simulink library "speedgoatlib_fpga_analog_io"  (R2024b)
settings: Solver=VariableStepAuto  StartTime=0.0  StopTime=10.0  RelTol=1e-3
undefined symbols (not defined in the file): IO336, sg_fpga_callBackInit_m_a1, sg_fpga_io324_analog_input_m, sg_fpga_io324_analog_output_m, sg_fpga_io324_analog_setup_m, sg_fpga_io325_analog_input_m, sg_fpga_io325_analog_output_m, sg_fpga_io325_analog_setup_m, sg_fpga_io334_analog_input_m, sg_fpga_io334_analog_output_m, sg_fpga_io334_analog_setup_m, sg_fpga_io336_analog_input_m, sg_fpga_io336_analog_output_m, sg_fpga_io336_analog_setup_m, sg_fpga_io337_analog_input_m, sg_fpga_io337_analog_output_m, sg_fpga_io337_analog_setup_m, sg_fpga_io3xx_120_analog_input_m, sg_fpga_io3xx_120_analog_output_m, sg_fpga_io3xx_120_analog_setup_m
(part 3 of 4)

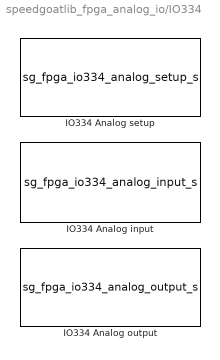
== system speedgoatlib_fpga_analog_io/IO334 ==
  IO334 Analog input : S-Function  InitFcn=sg_fpga_io334_analog_input_m.runInitFcn();  FunctionName=sg_fpga_io334_analog_input_s  Parameters=id, parSampleTime, parAiChannels, parAiChannelsStreamed, parAiReadPrevValue, parAiEnableFrame, parAiFrameSize  SFunctionDeploymentMode=off  EnableBusSupport=off  mask(ad_fpga_IO334){id=1, parSampleTime=-1, pciSlot=[-1,-1], parAiChannels=[1 2], parAiChannelsStreamed=[1 2], parAiReadPrevValue=0, parAiEnableFrame=0, parAdcCoupling=[1 1 1 1], parAdcContSampling=0, parAdcDmaEnable=0, parAdcActiveDmaDevices=[1 1 1 1], parAiFrameSize=100}
      mask prompts: id "Configurable I/O Module ID"; parSampleTime "Sample Time [s]"
      mask help: Speedgoat Driver Block<br>IO334-325k - IO334 Analog Input<br><br>&copy; 2007 - 2026, Speedgoat GmbH, <a href="matlab: web('www.speedgoat.com','-browser');">www.speedgoat.com</a>
      mask init:
      | sg_fpga_io334_analog_input_m.runMaskInit();
      mask Help: eval('sg.utils.help.show(''io_main/refentry_io334_analog_input_v1'');')
      mask TypeOptions id: 1 | 2 | 3 | 4 | 5 | 6 | 7 | 8 | 9 | 10
      mask Display: disp('Speedgoat\nIO334-325k\nAnalog input v1\nModule ID: 1');port_label('output',1,'1');port_label('output',2,'2');
  IO334 Analog output : S-Function  InitFcn=sg_fpga_io334_analog_output_m.runInitFcn();  FunctionName=sg_fpga_io334_analog_output_s  Parameters=id, parSampleTime, parAoChannels, parAoVoltageRange, parAoInitValues, parAoReset, parAoEnableFrame, parAoFrameSize  SFunctionDeploymentMode=off  EnableBusSupport=off  mask(da_fpga_IO334){id=1, parSampleTime=-1, pciSlot=[-1,-1], board=IO336-325k, parAoChannels=[1 3 5], parAoVoltageRange=[1 1 1], parDacOverRange=[0 0 0 0 0 0 0 0], parAoInitValues=[0 0 0], parAoReset=[1 1 1], parDacSyncOut=1, parAoEnableFrame=1, parDacActiveDmaDevices=[1 1 1 1], parDacDmaLatency=2, parAoFrameSize=1000}
      mask prompts: id "Configurable I/O Module ID"; parSampleTime "Sample Time [s]"
      mask help: Speedgoat Driver Block<br>IO334-325k - IO334 Analog Output<br><br>&copy; 2007 - 2026, Speedgoat GmbH, <a href="matlab: web('www.speedgoat.com','-browser');">www.speedgoat.com</a>
      mask init:
      | sg_fpga_io334_analog_output_m.runMaskInit();
      mask Help: eval('sg.utils.help.show(''io_main/refentry_io334_analog_output_v1'');')
      mask TypeOptions id: 1 | 2 | 3 | 4 | 5 | 6 | 7 | 8 | 9 | 10
      mask Display: disp('Speedgoat\nIO334-325k\nAnalog output v1\nModule ID: 1');port_label('input',1,'1');port_label('input',2,'3');port_label('input',3,'5');
  IO334 Analog setup : S-Function  InitFcn=sg_fpga_io334_analog_setup_m.runInitFcn();  FunctionName=sg_fpga_io334_analog_setup_s  Parameters=id, p.AdcActiveChannels, p.AdcFilterWidthPow2, p.AdcOversamplRate, p.AdcDisableSampleRead, parAdcAutoCorrection, p.AdcTriggerMode, p.AdcClockDivider, p.AdcInternalTrigger, p.AdcExternalTrigger, p.AdcEnableFrame, p.AdcFrameSize, p.DacChannels, p.DacVoltageRange, p.DacInitValues, p.DacReset, parDacAutoCorrection, p.DacTriggerMode, p.DacClockDivider, p.DacInternalTrigger, p.DacExternalTrigger, p.DacEnableFrame, p.DacFifoThreshold, p.DacSourceSelection, p.EnableTriggerForCm,p.DacUsesTimer  SFunctionModules=sg_fpga_analog_dma sg_AnalogInputCm_IO334 sg_AnalogOutputCm_IO334  SFunctionDeploymentMode=off  EnableBusSupport=off  mask(analog_setup_fpga_IO334){id=1, parEnableCodeModule1=off, parEnableCodeModule2=off, parEnableCodeModule3=off, parEnableCodeModule4=off, parEnableCodeModule5=off, parEnableCodeModule6=off, parEnableCodeModule7=off, parEnableCodeModule8=off, parAdcEnableIndividualTrigger=off, parAdcDisableSampleRead=off, parAdcTriggerMode1=Model Step, parAdcSampleRate1=1e5, parAdcDioTriggerChannel1=1, parAdcInternalTrigger1=<empty>, parAdcOversampling1=None, parAdcTriggerMode2=Model Step, parAdcSampleRate2=1e5, parAdcDioTriggerChannel2=1, parAdcInternalTrigger2=<empty>, parAdcOversampling2=None, parAdcTriggerMode3=Model Step, parAdcSampleRate3=1e5, parAdcDioTriggerChannel3=1, parAdcInternalTrigger3=<empty>, parAdcOversampling3=None, parAdcTriggerMode4=Model Step, parAdcSampleRate4=1e5, parAdcDioTriggerChannel4=1, parAdcInternalTrigger4=<empty>, parAdcOversampling4=None, parAdcTriggerMode5=Model Step, parAdcSampleRate5=1e5, parAdcDioTriggerChannel5=1, parAdcInternalTrigger5=<empty>, parAdcOversampling5=None, parAdcTriggerMode6=Model Step, parAdcSampleRate6=1e5, parAdcDioTriggerChannel6=1, parAdcInternalTrigger6=<empty>, parAdcOversampling6=None, parAdcTriggerMode7=Model Step, parAdcSampleRate7=1e5, parAdcDioTriggerChannel7=1, parAdcInternalTrigger7=<empty>, parAdcOversampling7=None, parAdcTriggerMode8=Model Step, parAdcSampleRate8=1e5, parAdcDioTriggerChannel8=1, parAdcInternalTrigger8=<empty>, parAdcOversampling8=None, parAdcReadPrevValueIndividualTrigger=off, parAdcEnableFrame=off, parAdcTriggerMode=Model Step, parAdcReadPrevValue=on, parAdcSampleRate=100e3, parAdcDioTriggerChannel=1, parAdcInternalTrigger=<empty>, parAdcOversampling=None, parAdcTriggerResolution=1e-08, parAdcSampleRateFrame=1e5, parAdcFrameSize=100, parAdcSampleTime=-1, parDacTriggerMode=Model Step, parDacInternalTrigger=<empty>, parDacDioTriggerChannel=1, parDacEnableFrame=off, dacUsesTimer=off, parDacFifoThreshold=100, parDacTriggerResolution=1e-08, parDacSampleRate=1e6, parDacFrameSize=1000, parDacSampleTime=-1, parAdcChannel1=on, parAdcChannel2=on, parAdcChannel3=off, parAdcChannel4=off, parAdcChannel5=off, parAdcChannel6=off, parAdcChannel7=off, parAdcChannel8=off, parAdcChannel9=off, parAdcChannel10=off, parAdcChannel11=off, parAdcChannel12=off, parAdcChannel13=off, parAdcChannel14=off, parAdcChannel15=off, parAdcChannel16=off, parAdcAutoCorrection=on, parDacChannel1=on, parDacChannel2=on, parDacChannel3=off, parDacChannel4=off, parDacChannel5=off, parDacChannel6=off, parDacChannel7=off, parDacChannel8=off, parDacChannel9=off, parDacChannel10=off, parDacChannel11=off, parDacChannel12=off, parDacChannel13=off, parDacChannel14=off, parDacChannel15=off, parDacChannel16=off, parDacRange1=+-10 V, parDacInitValue1=0, parDacReset1=on, parDacRange2=+-10 V, parDacInitValue2=0, parDacReset2=on, parDacRange3=+-10 V, parDacInitValue3=0, parDacReset3=on, parDacRange4=+-10 V, parDacInitValue4=0, parDacReset4=on, parDacRange5=+-10 V, parDacInitValue5=0, parDacReset5=on, parDacRange6=+-10 V, parDacInitValue6=0, parDacReset6=on, parDacRange7=+-10 V, parDacInitValue7=0, parDacReset7=on, parDacRange8=+-10 V, parDacInitValue8=0, parDacReset8=on, parDacRange9=+-10 V, parDacInitValue9=0, parDacReset9=on, parDacRange10=+-10 V, parDacInitValue10=0, parDacReset10=on, parDacRange11=+-10 V, parDacInitValue11=0, parDacReset11=on, parDacRange12=+-10 V, parDacInitValue12=0, parDacReset12=on, parDacRange13=+-10 V, parDacInitValue13=0, parDacReset13=on, parDacRange14=+-10 V, parDacInitValue14=0, parDacReset14=on, parDacRange15=+-10 V, parDacInitValue15=0, parDacReset15=on, parDacRange16=+-10 V, parDacInitValue16=0, parDacReset16=on, parDacAutoCorrection=on}
      mask prompts: id "Configurable I/O Module ID"; parAdcEnableIndividualTrigger "Enable Individual Trigger Settings"; parAdcDisableSampleRead "Disable Sample and Read"; parAdcTriggerMode1 "ADC Sample Trigger"; parAdcSampleRate1 "ADC Sample Rate [Hz]"; parAdcDioTriggerChannel1 "Digital I/O Channel"; parAdcInternalTrigger1 "Internal Signal"; parAdcOversampling1 "Oversampling Factor"; parAdcTriggerMode2 "ADC Sample Trigger"; parAdcSampleRate2 "ADC Sample Rate [Hz]"; parAdcDioTriggerChannel2 "Digital I/O Channel"; parAdcInternalTrigger2 "Internal Signal"; parAdcOversampling2 "Oversampling Factor"; parAdcTriggerMode3 "ADC Sample Trigger"; parAdcSampleRate3 "ADC Sample Rate [Hz]"; parAdcDioTriggerChannel3 "Digital I/O Channel"; parAdcInternalTrigger3 "Internal Signal"; parAdcOversampling3 "Oversampling Factor"; parAdcTriggerMode4 "ADC Sample Trigger"; parAdcSampleRate4 "ADC Sample Rate [Hz]"; parAdcDioTriggerChannel4 "Digital I/O Channel"; parAdcInternalTrigger4 "Internal Signal"; parAdcOversampling4 "Oversampling Factor"; parAdcTriggerMode5 "ADC Sample Trigger"; parAdcSampleRate5 "ADC Sample Rate [Hz]"; parAdcDioTriggerChannel5 "Digital I/O Channel"; parAdcInternalTrigger5 "Internal Signal"; parAdcOversampling5 "Oversampling Factor"; parAdcTriggerMode6 "ADC Sample Trigger"; parAdcSampleRate6 "ADC Sample Rate [Hz]"; parAdcDioTriggerChannel6 "Digital I/O Channel"; parAdcInternalTrigger6 "Internal Signal"; parAdcOversampling6 "Oversampling Factor"; parAdcTriggerMode7 "ADC Sample Trigger"; parAdcSampleRate7 "ADC Sample Rate [Hz]"; parAdcDioTriggerChannel7 "Digital I/O Channel"; parAdcInternalTrigger7 "Internal Signal"; parAdcOversampling7 "Oversampling Factor"; parAdcTriggerMode8 "ADC Sample Trigger"; parAdcSampleRate8 "ADC Sample Rate [Hz]"; parAdcDioTriggerChannel8 "Digital I/O Channel"; parAdcInternalTrigger8 "Internal Signal"; parAdcOversampling8 "Oversampling Factor"; parAdcReadPrevValueIndividualTrigger "Read Value From Previous Model Step"; parAdcEnableFrame "Enable DMA Interrupt"; parAdcTriggerMode "ADC Sample Trigger"; parAdcReadPrevValue "Read Value From Previous Model Step"; parAdcSampleRate "ADC Sample Rate [Hz]"; parAdcDioTriggerChannel "Digital I/O Channel"; parAdcInternalTrigger "Internal Signal"; parAdcOversampling "Oversampling Factor"; parAdcTriggerResolution "Trigger Resolution [s]"; parAdcSampleRateFrame "ADC Sample Rate [Hz]"; parAdcFrameSize "Frame Size (samples/channel)"; parAdcSampleTime "Input Block Sample Time [s]"; parDacTriggerMode "DAC Sample Trigger"; parDacInternalTrigger "Internal Signal"; parDacDioTriggerChannel "Digital I/O Channel"; parDacEnableFrame "Enable DMA Interrupt"; dacUsesTimer "Set Sampling Frequency"; parDacFifoThreshold "FIFO Threshold (samples/channel)"; parDacTriggerResolution "Trigger Resolution [s]"; parDacSampleRate "DAC Sample Rate [Hz]"; parDacFrameSize "Frame Size (samples/channel)"; parDacSampleTime "Output Block Sample Time [s]"; parAdcChannel1 "Ch 01"; parAdcChannel2 "Ch 02"; parAdcChannel3 "Ch 03"; parAdcChannel4 "Ch 04"; parAdcChannel5 "Ch 05"; parAdcChannel6 "Ch 06"; parAdcChannel7 "Ch 07"; parAdcChannel8 "Ch 08"; parAdcChannel9 "Ch 09"; parAdcChannel10 "Ch 10"; parAdcChannel11 "Ch 11"; parAdcChannel12 "Ch 12"; parAdcChannel13 "Ch 13"; parAdcChannel14 "Ch 14"; parAdcChannel15 "Ch 15"; parAdcChannel16 "Ch 16"; parAdcAutoCorrection "Automatic Data Correction (for Debugging)"; parDacChannel1 "Ch 1"; parDacChannel2 "Ch 2"; parDacChannel3 "Ch 3"; parDacChannel4 "Ch 4"; parDacChannel5 "Ch 5"; parDacChannel6 "Ch 6"; parDacChannel7 "Ch 7"; parDacChannel8 "Ch 8"; parDacChannel9 "Ch 9"; parDacChannel10 "Ch 10"; parDacChannel11 "Ch 11"; parDacChannel12 "Ch 12"; parDacChannel13 "Ch 13"; parDacChannel14 "Ch 14"; parDacChannel15 "Ch 15"; parDacChannel16 "Ch 16"; parDacRange1 "Output Range"; parDacInitValue1 "Initial Value [V]"; parDacReset1 "Reset to Initial Value"; parDacRange2 "Output Range"; parDacInitValue2 "Initial Value [V]"; parDacReset2 "Reset to Initial Value"; parDacRange3 "Output Range"; parDacInitValue3 "Initial Value [V]"; parDacReset3 "Reset to Initial Value"; parDacRange4 "Output Range"; parDacInitValue4 "Initial Value [V]"; parDacReset4 "Reset to Initial Value"; parDacRange5 "Output Range"; parDacInitValue5 "Initial Value [V]"; parDacReset5 "Reset to Initial Value"; parDacRange6 "Output Range"; parDacInitValue6 "Initial Value [V]"; parDacReset6 "Reset to Initial Value"; parDacRange7 "Output Range"; parDacInitValue7 "Initial Value [V]"; parDacReset7 "Reset to Initial Value"; parDacRange8 "Output Range"; parDacInitValue8 "Initial Value [V]"; parDacReset8 "Reset to Initial Value"; parDacRange9 "Output Range"; parDacInitValue9 "Initial Value [V]"; parDacReset9 "Reset to Initial Value"; parDacRange10 "Output Range"; parDacInitValue10 "Initial Value [V]"; parDacReset10 "Reset to Initial Value"; parDacRange11 "Output Range"; parDacInitValue11 "Initial Value [V]"; parDacReset11 "Reset to Initial Value"; parDacRange12 "Output Range"; parDacInitValue12 "Initial Value [V]"; parDacReset12 "Reset to Initial Value"; parDacRange13 "Output Range"; parDacInitValue13 "Initial Value [V]"; parDacReset13 "Reset to Initial Value"; parDacRange14 "Output Range"; parDacInitValue14 "Initial Value [V]"; parDacReset14 "Reset to Initial Value"; parDacRange15 "Output Range"; parDacInitValue15 "Initial Value [V]"; parDacReset15 "Reset to Initial Value"; parDacRange16 "Output Range"; parDacInitValue16 "Initial Value [V]"; parDacReset16 "Reset to Initial Value"; parDacAutoCorrection "Automatic Data Correction (for Debugging)"
      mask help: Speedgoat Driver Block<br>IO334-325k - IO334 Analog setup<br><br>&copy; 2007 - 2026, Speedgoat GmbH, <a href="matlab: web('www.speedgoat.com','-browser');">www.speedgoat.com</a>
      mask init:
      | p = sg_fpga_io334_analog_setup_m.runMaskInit();
      settings: OpenFcn=sg_fpga_io334_analog_setup_m.runOpenMaskCb();
      mask Help: eval('sg.utils.help.show(''io_main/refentry_io334_analog_setup_v1'');')
      mask TypeOptions id: 1 | 2 | 3 | 4 | 5 | 6 | 7 | 8 | 9 | 10
      mask Callback parEnableCodeModule1: sg_fpga_io334_analog_setup_m.runEnableCmCb(1);
      mask Callback parEnableCodeModule2: sg_fpga_io334_analog_setup_m.runEnableCmCb(2);
      mask Callback parEnableCodeModule3: sg_fpga_io334_analog_setup_m.runEnableCmCb(3);
      mask Callback parEnableCodeModule4: sg_fpga_io334_analog_setup_m.runEnableCmCb(4);
      mask Callback parEnableCodeModule5: sg_fpga_io334_analog_setup_m.runEnableCmCb(5);
      mask Callback parEnableCodeModule6: sg_fpga_io334_analog_setup_m.runEnableCmCb(6);
      mask Callback parEnableCodeModule7: sg_fpga_io334_analog_setup_m.runEnableCmCb(7);
      mask Callback parEnableCodeModule8: sg_fpga_io334_analog_setup_m.runEnableCmCb(8);
      mask Callback parAdcEnableIndividualTrigger: sg_fpga_io334_analog_setup_m.runAnalogInputCb();
      mask Callback parAdcDisableSampleRead: sg_fpga_io334_analog_setup_m.runAnalogInputCb();
      mask TypeOptions parAdcTriggerMode1: Model Step | I/O Module Clock | I/O Module Internal Signal | I/O Module Digital I/O
      mask Callback parAdcTriggerMode1: sg_fpga_io334_analog_setup_m.runAdcTriggerCb('suffix', '1');
      mask TypeOptions parAdcInternalTrigger1: <empty>
      mask TypeOptions parAdcOversampling1: None | 2 | 4 | 8 | 16 | 32 | 64
      mask TypeOptions parAdcTriggerMode2: Model Step | I/O Module Clock | I/O Module Internal Signal | I/O Module Digital I/O
      mask Callback parAdcTriggerMode2: sg_fpga_io334_analog_setup_m.runAdcTriggerCb('suffix', '2');
      mask TypeOptions parAdcInternalTrigger2: <empty>
      mask TypeOptions parAdcOversampling2: None | 2 | 4 | 8 | 16 | 32 | 64
      mask TypeOptions parAdcTriggerMode3: Model Step | I/O Module Clock | I/O Module Internal Signal | I/O Module Digital I/O
      mask Callback parAdcTriggerMode3: sg_fpga_io334_analog_setup_m.runAdcTriggerCb('suffix', '3');
      mask TypeOptions parAdcInternalTrigger3: <empty>
      mask TypeOptions parAdcOversampling3: None | 2 | 4 | 8 | 16 | 32 | 64
      mask TypeOptions parAdcTriggerMode4: Model Step | I/O Module Clock | I/O Module Internal Signal | I/O Module Digital I/O
      mask Callback parAdcTriggerMode4: sg_fpga_io334_analog_setup_m.runAdcTriggerCb('suffix', '4');
      mask TypeOptions parAdcInternalTrigger4: <empty>
      mask TypeOptions parAdcOversampling4: None | 2 | 4 | 8 | 16 | 32 | 64
      mask TypeOptions parAdcTriggerMode5: Model Step | I/O Module Clock | I/O Module Internal Signal | I/O Module Digital I/O
      mask Callback parAdcTriggerMode5: sg_fpga_io334_analog_setup_m.runAdcTriggerCb('suffix', '5');
      mask TypeOptions parAdcInternalTrigger5: <empty>
      mask TypeOptions parAdcOversampling5: None | 2 | 4 | 8 | 16 | 32 | 64
      mask TypeOptions parAdcTriggerMode6: Model Step | I/O Module Clock | I/O Module Internal Signal | I/O Module Digital I/O
      mask Callback parAdcTriggerMode6: sg_fpga_io334_analog_setup_m.runAdcTriggerCb('suffix', '6');
      mask TypeOptions parAdcInternalTrigger6: <empty>
      mask TypeOptions parAdcOversampling6: None | 2 | 4 | 8 | 16 | 32 | 64
      mask TypeOptions parAdcTriggerMode7: Model Step | I/O Module Clock | I/O Module Internal Signal | I/O Module Digital I/O
      mask Callback parAdcTriggerMode7: sg_fpga_io334_analog_setup_m.runAdcTriggerCb('suffix', '7');
      mask TypeOptions parAdcInternalTrigger7: <empty>
      mask TypeOptions parAdcOversampling7: None | 2 | 4 | 8 | 16 | 32 | 64
      mask TypeOptions parAdcTriggerMode8: Model Step | I/O Module Clock | I/O Module Internal Signal | I/O Module Digital I/O
      mask Callback parAdcTriggerMode8: sg_fpga_io334_analog_setup_m.runAdcTriggerCb('suffix', '8');
      mask TypeOptions parAdcInternalTrigger8: <empty>
      mask TypeOptions parAdcOversampling8: None | 2 | 4 | 8 | 16 | 32 | 64
      mask Callback parAdcEnableFrame: sg_fpga_io334_analog_setup_m.runEnableFrameCb();
      mask TypeOptions parAdcTriggerMode: Model Step | I/O Module Clock | I/O Module Internal Signal | I/O Module Digital I/O
      mask Callback parAdcTriggerMode: sg_fpga_io334_analog_setup_m.runAdcTriggerCb();
      mask TypeOptions parAdcInternalTrigger: <empty>
      mask TypeOptions parAdcOversampling: None | 2 | 4 | 8 | 16 | 32 | 64
      mask TypeOptions parDacTriggerMode: Model Step | I/O Module Clock | I/O Module Internal Signal | I/O Module Digital I/O
      mask Callback parDacTriggerMode: sg_fpga_io334_analog_setup_m.runDacTriggerCb();
      mask TypeOptions parDacInternalTrigger: <empty>
      mask Callback parDacEnableFrame: sg_fpga_io334_analog_setup_m.runDacTriggerCb();
      mask Callback dacUsesTimer: sg_fpga_io334_analog_setup_m.runDacTriggerCb();
      mask Callback parAdcChannel1: sg_fpga_io334_analog_setup_m.runAnalogInputCb();
      mask Callback parAdcChannel2: sg_fpga_io334_analog_setup_m.runAnalogInputCb();
      mask Callback parAdcChannel3: sg_fpga_io334_analog_setup_m.runAnalogInputCb();
      mask Callback parAdcChannel4: sg_fpga_io334_analog_setup_m.runAnalogInputCb();
      mask Callback parAdcChannel5: sg_fpga_io334_analog_setup_m.runAnalogInputCb();
      mask Callback parAdcChannel6: sg_fpga_io334_analog_setup_m.runAnalogInputCb();
      mask Callback parAdcChannel7: sg_fpga_io334_analog_setup_m.runAnalogInputCb();
      mask Callback parAdcChannel8: sg_fpga_io334_analog_setup_m.runAnalogInputCb();
      mask Callback parAdcChannel9: sg_fpga_io334_analog_setup_m.runAnalogInputCb();
      mask Callback parAdcChannel10: sg_fpga_io334_analog_setup_m.runAnalogInputCb();
      mask Callback parAdcChannel11: sg_fpga_io334_analog_setup_m.runAnalogInputCb();
      mask Callback parAdcChannel12: sg_fpga_io334_analog_setup_m.runAnalogInputCb();
      mask Callback parAdcChannel13: sg_fpga_io334_analog_setup_m.runAnalogInputCb();
      mask Callback parAdcChannel14: sg_fpga_io334_analog_setup_m.runAnalogInputCb();
      mask Callback parAdcChannel15: sg_fpga_io334_analog_setup_m.runAnalogInputCb();
      mask Callback parAdcChannel16: sg_fpga_io334_analog_setup_m.runAnalogInputCb();
      mask Callback parDacChannel1: sg_fpga_io334_analog_setup_m.runAnalogOutputCb();
      mask Callback parDacChannel2: sg_fpga_io334_analog_setup_m.runAnalogOutputCb();
      mask Callback parDacChannel3: sg_fpga_io334_analog_setup_m.runAnalogOutputCb();
      mask Callback parDacChannel4: sg_fpga_io334_analog_setup_m.runAnalogOutputCb();
      mask Callback parDacChannel5: sg_fpga_io334_analog_setup_m.runAnalogOutputCb();
      mask Callback parDacChannel6: sg_fpga_io334_analog_setup_m.runAnalogOutputCb();
      mask Callback parDacChannel7: sg_fpga_io334_analog_setup_m.runAnalogOutputCb();
      mask Callback parDacChannel8: sg_fpga_io334_analog_setup_m.runAnalogOutputCb();
      mask Callback parDacChannel9: sg_fpga_io334_analog_setup_m.runAnalogOutputCb();
      mask Callback parDacChannel10: sg_fpga_io334_analog_setup_m.runAnalogOutputCb();
      mask Callback parDacChannel11: sg_fpga_io334_analog_setup_m.runAnalogOutputCb();
      mask Callback parDacChannel12: sg_fpga_io334_analog_setup_m.runAnalogOutputCb();
      mask Callback parDacChannel13: sg_fpga_io334_analog_setup_m.runAnalogOutputCb();
      mask Callback parDacChannel14: sg_fpga_io334_analog_setup_m.runAnalogOutputCb();
      mask Callback parDacChannel15: sg_fpga_io334_analog_setup_m.runAnalogOutputCb();
      mask Callback parDacChannel16: sg_fpga_io334_analog_setup_m.runAnalogOutputCb();
      mask TypeOptions parDacRange1: +-2.5 V | +-5 V | +-10 V
      mask TypeOptions parDacRange2: +-2.5 V | +-5 V | +-10 V
      mask TypeOptions parDacRange3: +-2.5 V | +-5 V | +-10 V
      mask TypeOptions parDacRange4: +-2.5 V | +-5 V | +-10 V
      mask TypeOptions parDacRange5: +-2.5 V | +-5 V | +-10 V
      mask TypeOptions parDacRange6: +-2.5 V | +-5 V | +-10 V
      mask TypeOptions parDacRange7: +-2.5 V | +-5 V | +-10 V
      mask TypeOptions parDacRange8: +-2.5 V | +-5 V | +-10 V
      mask TypeOptions parDacRange9: +-2.5 V | +-5 V | +-10 V
      mask TypeOptions parDacRange10: +-2.5 V | +-5 V | +-10 V
      mask TypeOptions parDacRange11: +-2.5 V | +-5 V | +-10 V
      mask TypeOptions parDacRange12: +-2.5 V | +-5 V | +-10 V
      mask TypeOptions parDacRange13: +-2.5 V | +-5 V | +-10 V
      mask TypeOptions parDacRange14: +-2.5 V | +-5 V | +-10 V
      mask TypeOptions parDacRange15: +-2.5 V | +-5 V | +-10 V
      mask TypeOptions parDacRange16: +-2.5 V | +-5 V | +-10 V
      mask DialogControl tabMain Prompt: Main
      mask DialogControl boxModuleSettings Prompt: Module Settings
      mask DialogControl boxCodeModules Prompt: Code Module Functionality
      mask DialogControl boxAdcTrigger Prompt: Analog Input Settings
      mask DialogControl boxAdcIndividualTrigger Prompt: Individual Trigger Settings (Sample Based)
      mask DialogControl boxAdcTrigger1 Prompt: Channel 01-02
      mask DialogControl boxAdcTrigger2 Prompt: Channel 03-04
      mask DialogControl boxAdcTrigger3 Prompt: Channel 05-06
      mask DialogControl boxAdcTrigger4 Prompt: Channel 07-08
      mask DialogControl boxAdcTrigger5 Prompt: Channel 09-10
      mask DialogControl boxAdcTrigger6 Prompt: Channel 11-12
      mask DialogControl boxAdcTrigger7 Prompt: Channel 13-14
      mask DialogControl boxAdcTrigger8 Prompt: Channel 15-16
      mask DialogControl boxAdcCommonTrigger Prompt: Common Trigger Settings
      mask DialogControl boxAdcFrameSettings Prompt: Frame-Based Settings
      mask DialogControl parAdcTriggerResolutionInfo Prompt: placeholder
      mask DialogControl parAdcSampleRateFrameInfo Prompt:
      | => 100 kHz
      | (10 us/sample)
      mask DialogControl parAdcFrameSizeInfo Prompt: => 100
      mask DialogControl parAdcSampleTimeInfo Prompt: => -1 s
      mask DialogControl boxDacTrigger Prompt: Analog Output Trigger
      mask DialogControl boxDacFrameSettings Prompt: Update Settings
      mask DialogControl parDacFifoThresholdInfo Prompt: placeholder
      mask DialogControl parDacTriggerResolutionInfo Prompt: placeholder
      mask DialogControl parDacSampleRateInfo Prompt:
      | => 8.33333 MHz
      | (120 ns/sample)
      mask DialogControl parDacFrameSizeInfo Prompt: => 1000
      mask DialogControl parDacSampleTimeInfo Prompt: => 120 us
      mask DialogControl tabAdc Prompt: Analog Inputs
      mask DialogControl boxAdc1 Prompt: Channel 01-08
      mask DialogControl boxAdc2 Prompt: Channel 09-16
      mask DialogControl tabDac Prompt: Analog Outputs
      mask DialogControl boxDacSetting Prompt: Channel Settings
      mask DialogControl boxAoChannels Prompt: Available Channels
      mask DialogControl boxDacChannel1 Prompt: Channel 1
      mask DialogControl boxDacChannel2 Prompt: Channel 2
      mask DialogControl boxDacChannel3 Prompt: Channel 3
      mask DialogControl boxDacChannel4 Prompt: Channel 4
      mask DialogControl boxDacChannel5 Prompt: Channel 5
      mask DialogControl boxDacChannel6 Prompt: Channel 6
      mask DialogControl boxDacChannel7 Prompt: Channel 7
      mask DialogControl boxDacChannel8 Prompt: Channel 8
      mask DialogControl boxDacChannel9 Prompt: Channel 9
      mask DialogControl boxDacChannel10 Prompt: Channel 10
      mask DialogControl boxDacChannel11 Prompt: Channel 11
      mask DialogControl boxDacChannel12 Prompt: Channel 12
      mask DialogControl boxDacChannel13 Prompt: Channel 13
      mask DialogControl boxDacChannel14 Prompt: Channel 14
      mask DialogControl boxDacChannel15 Prompt: Channel 15
      mask DialogControl boxDacChannel16 Prompt: Channel 16
      mask Display: disp('Speedgoat\nIO334-325k\nAnalog setup v1\nModule ID: 1');

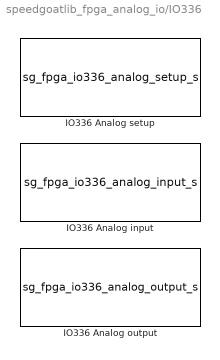
== system speedgoatlib_fpga_analog_io/IO336 ==
  IO336 Analog input : S-Function  InitFcn=sg_fpga_io336_analog_input_m.runInitFcn();  FunctionName=sg_fpga_io336_analog_input_s  Parameters=id, parSampleTime, parAiChannels, parAiChannelsStreamed, parAiVoltageRange, parAiTriggerMode, parAiReadPrevValue, parAiEnableFrame, parAiFrameSize  SFunctionDeploymentMode=off  EnableBusSupport=off  mask(ad_fpga_IO336){id=1, parSampleTime=-1, pciSlot=[-1,-1], parAiChannels=[1 2], parAiChannelsStreamed=[1 2], parAiTriggerMode=[2 2], parAiReadPrevValue=0, parAiEnableFrame=0, parAiVoltageRange=[0 3 3 3 3 3 3 3], parAdcCoupling=[1 1 1 1], parAdcContSampling=0, parAdcDmaEnable=0, parAdcActiveDmaDevices=[1 1 1 1], parAiFrameSize=100}
      mask prompts: id "Configurable I/O Module ID"; parSampleTime "Sample Time [s]"
      mask help: Speedgoat Driver Block<br>IO336-325k - IO336 Analog Input<br><br>&copy; 2007 - 2026, Speedgoat GmbH, <a href="matlab: web('www.speedgoat.com','-browser');">www.speedgoat.com</a>
      mask init:
      | sg_fpga_io336_analog_input_m.runMaskInit();
      mask Help: eval('sg.utils.help.show(''io_main/refentry_io336_analog_input_v1'');')
      mask TypeOptions id: 1 | 2 | 3 | 4 | 5 | 6 | 7 | 8 | 9 | 10
      mask Display: disp('Speedgoat\nIO336-325k\nAnalog input v1\nModule ID: 1');port_label('output',1,'1');port_label('output',2,'2');
  IO336 Analog output : S-Function  InitFcn=sg_fpga_io336_analog_output_m.runInitFcn();  FunctionName=sg_fpga_io336_analog_output_s  Parameters=id, parSampleTime, parAoChannels, parAoVoltageRange, parAoInitValues, parAoReset, parAoEnableFrame, parAoFrameSize  SFunctionDeploymentMode=off  EnableBusSupport=off  mask(da_fpga_IO336){id=1, parSampleTime=-1, pciSlot=[-1,-1], board=IO336-325k, parAoChannels=[1 2], parAoVoltageRange=[1 1], parDacOverRange=[0 0 0 0 0 0 0 0], parAoInitValues=[0 0], parAoReset=[1 1], parDacSyncOut=1, parAoEnableFrame=0, parDacActiveDmaDevices=[1 1 1 1], parDacDmaLatency=2, parAoFrameSize=1000}
      mask prompts: id "Configurable I/O Module ID"; parSampleTime "Sample Time [s]"
      mask help: Speedgoat Driver Block<br>IO336-325k - IO336 Analog Output<br><br>&copy; 2007 - 2026, Speedgoat GmbH, <a href="matlab: web('www.speedgoat.com','-browser');">www.speedgoat.com</a>
      mask init:
      | sg_fpga_io336_analog_output_m.runMaskInit();
      mask Help: eval('sg.utils.help.show(''io_main/refentry_io336_analog_output_v1'');')
      mask TypeOptions id: 1 | 2 | 3 | 4 | 5 | 6 | 7 | 8 | 9 | 10
      mask Display: disp('Speedgoat\nIO336-325k\nAnalog output v1\nModule ID: 1');port_label('input',1,'1');port_label('input',2,'2');
  IO336 Analog setup : S-Function  InitFcn=sg_fpga_io336_analog_setup_m.runInitFcn();  FunctionName=sg_fpga_io336_analog_setup_s  Parameters=id, p.AdcActiveChannels, p.AdcVoltageRange, p.AdcFilterWidthPow2, p.AdcOversamplRate, parAdcAutoCorrection, p.AdcTriggerMode, p.AdcClockDivider, p.AdcInternalTrigger, p.AdcExternalTrigger, p.AdcEnableFrame, p.AdcFrameSize, p.DacChannels, p.DacVoltageRange, p.DacInitValues, p.DacReset, parDacAutoCorrection, p.DacTriggerMode, p.DacClockDivider, p.DacInternalTrigger, p.DacExternalTrigger, p.DacEnableFrame, p.DacFifoThreshold, p.DacSourceSelection, p.EnableTriggerForCm,p.DacUsesTimer  SFunctionModules=sg_fpga_analog_dma sg_AnalogInputCm_IO336 sg_AnalogOutputCm  SFunctionDeploymentMode=off  EnableBusSupport=off  mask(analog_setup_fpga_IO336){id=1, parEnableCodeModule1=off, parEnableCodeModule2=off, parEnableCodeModule3=off, parEnableCodeModule4=off, parEnableCodeModule5=off, parEnableCodeModule6=off, parEnableCodeModule7=off, parEnableCodeModule8=off, parAdcEnableIndividualTrigger=off, parAdcTriggerMode1=Model Step, parAdcSampleRate1=0, parAdcDioTriggerChannel1=1, parAdcInternalTrigger1=<empty>, parAdcOversampling1=None, parAdcTriggerMode2=Model Step, parAdcSampleRate2=0, parAdcDioTriggerChannel2=1, parAdcInternalTrigger2=<empty>, parAdcOversampling2=None, parAdcReadPrevValueIndividualTrigger=off, parAdcEnableFrame=off, parAdcTriggerMode=I/O Module Clock, parAdcReadPrevValue=on, parAdcSampleRate=100e3, parAdcDioTriggerChannel=1, parAdcInternalTrigger=<empty>, parAdcOversampling=None, parAdcTriggerResolution=1e-08, parAdcSampleRateFrame=100e3, parAdcFrameSize=100, parAdcSampleTime=-1, parDacTriggerMode=I/O Module Clock, parDacInternalTrigger=<empty>, parDacDioTriggerChannel=0, parDacEnableFrame=on, dacUsesTimer=on, parDacFifoThreshold=100, parDacTriggerResolution=1e-08, parDacSampleRate=1e6, parDacFrameSize=1000, parDacSampleTime=-1, parAdcChannel1=on, parAdcChannel2=on, parAdcChannel3=off, parAdcChannel4=off, parAdcChannel5=off, parAdcChannel6=off, parAdcChannel7=off, parAdcChannel8=off, parVoltageRangePerChannelEn1=off, parAdcRangeAll1=+/- 20V, parAdcRange1=+/- 20V, parAdcRange3=+/- 20V, parAdcRange2=+/- 20V, parAdcRange4=+/- 20V, parAdcChannel9=off, parAdcChannel10=off, parAdcChannel11=off, parAdcChannel12=off, parAdcChannel13=off, parAdcChannel14=off, parAdcChannel15=off, parAdcChannel16=off, parVoltageRangePerChannelEn2=off, parAdcRangeAll2=+/- 20V, parAdcRange5=+/- 20V, parAdcRange7=+/- 20V, parAdcRange6=+/- 20V, parAdcRange8=+/- 20V, parAdcAutoCorrection=on, parDacChannel1=on, parDacChannel2=on, parDacChannel3=off, parDacChannel4=off, parDacChannel5=off, parDacChannel6=off, parDacChannel7=off, parDacChannel8=off, parDacRange1=+-10 V, parDacInitValue1=0, parDacReset1=on, parDacRange2=+-10 V, parDacInitValue2=0, parDacReset2=on, parDacRange3=+-10 V, parDacInitValue3=0, parDacReset3=on, parDacRange4=+-10 V, parDacInitValue4=0, parDacReset4=on, parDacRange5=+-10 V, parDacInitValue5=0, parDacReset5=on, parDacRange6=+-10 V, parDacInitValue6=0, parDacReset6=on, parDacRange7=+-10 V, parDacInitValue7=0, parDacReset7=on, parDacRange8=+-10 V, parDacInitValue8=0, parDacReset8=on, parDacAutoCorrection=on}
      mask prompts: id "Configurable I/O Module ID"; parAdcEnableIndividualTrigger "Enable Individual Trigger Settings"; parAdcTriggerMode1 "ADC Sample Trigger"; parAdcSampleRate1 "ADC Sample Rate [Hz]"; parAdcDioTriggerChannel1 "Digital I/O Channel"; parAdcInternalTrigger1 "Internal Signal"; parAdcOversampling1 "Oversampling Factor"; parAdcTriggerMode2 "ADC Sample Trigger"; parAdcSampleRate2 "ADC Sample Rate [Hz]"; parAdcDioTriggerChannel2 "Digital I/O Channel"; parAdcInternalTrigger2 "Internal Signal"; parAdcOversampling2 "Oversampling Factor"; parAdcReadPrevValueIndividualTrigger "Read Value From Previous Model Step"; parAdcEnableFrame "Enable DMA Interrupt"; parAdcTriggerMode "ADC Sample Trigger"; parAdcReadPrevValue "Read Value From Previous Model Step"; parAdcSampleRate "ADC Sample Rate [Hz]"; parAdcDioTriggerChannel "Digital I/O Channel"; parAdcInternalTrigger "Internal Signal"; parAdcOversampling "Oversampling Factor"; parAdcTriggerResolution "Trigger Resolution [s]"; parAdcSampleRateFrame "ADC Sample Rate [Hz]"; parAdcFrameSize "Frame Size (samples/channel)"; parAdcSampleTime "Input Block Sample Time [s]"; parDacTriggerMode "DAC Sample Trigger"; parDacInternalTrigger "Internal Signal"; parDacDioTriggerChannel "Digital I/O Channel"; parDacEnableFrame "Enable DMA Interrupt"; dacUsesTimer "Set Sampling Frequency"; parDacFifoThreshold "FIFO Threshold (samples/channel)"; parDacTriggerResolution "Trigger resolution [s]"; parDacSampleRate "DAC Sample Rate [Hz]"; parDacFrameSize "Frame Size (samples/channel)"; parDacSampleTime "Output Block Sample Time [s]"; parAdcChannel1 "Ch 01"; parAdcChannel2 "Ch 02"; parAdcChannel3 "Ch 03"; parAdcChannel4 "Ch 04"; parAdcChannel5 "Ch 05"; parAdcChannel6 "Ch 06"; parAdcChannel7 "Ch 07"; parAdcChannel8 "Ch 08"; parVoltageRangePerChannelEn1 "Set Voltage Range per Channel Pair"; parAdcRangeAll1 "Voltage Range"; parAdcRange1 "Ch 01 / 02"; parAdcRange3 "Ch 05 / 06"; parAdcRange2 "Ch 03 / 04"; parAdcRange4 "Ch 07 / 08"; parAdcChannel9 "Ch 09"; parAdcChannel10 "Ch 10"; parAdcChannel11 "Ch 11"; parAdcChannel12 "Ch 12"; parAdcChannel13 "Ch 13"; parAdcChannel14 "Ch 14"; parAdcChannel15 "Ch 15"; parAdcChannel16 "Ch 16"; parVoltageRangePerChannelEn2 "Set Voltage Range per Channel Pair"; parAdcRangeAll2 "Voltage Range"; parAdcRange5 "Ch 09 / 10"; parAdcRange7 "Ch 13 / 14"; parAdcRange6 "Ch 11 / 12"; parAdcRange8 "Ch 15 / 16"; parAdcAutoCorrection "Automatic Data Correction (for Debugging)"; parDacChannel1 "Ch 1"; parDacChannel2 "Ch 2"; parDacChannel3 "Ch 3"; parDacChannel4 "Ch 4"; parDacChannel5 "Ch 5"; parDacChannel6 "Ch 6"; parDacChannel7 "Ch 7"; parDacChannel8 "Ch 8"; parDacRange1 "Output Range"; parDacInitValue1 "Initial Value [V]"; parDacReset1 "Reset to Initial Value"; parDacRange2 "Output Range"; parDacInitValue2 "Initial Value [V]"; parDacReset2 "Reset to Initial Value"; parDacRange3 "Output Range"; parDacInitValue3 "Initial Value [V]"; parDacReset3 "Reset to Initial Value"; parDacRange4 "Output Range"; parDacInitValue4 "Initial Value [V]"; parDacReset4 "Reset to Initial Value"; parDacRange5 "Output Range"; parDacInitValue5 "Initial Value [V]"; parDacReset5 "Reset to Initial Value"; parDacRange6 "Output Range"; parDacInitValue6 "Initial Value [V]"; parDacReset6 "Reset to Initial Value"; parDacRange7 "Output Range"; parDacInitValue7 "Initial Value [V]"; parDacReset7 "Reset to Initial Value"; parDacRange8 "Output Range"; parDacInitValue8 "Initial Value [V]"; parDacReset8 "Reset to Initial Value"; parDacAutoCorrection "Automatic Data Correction (for Debugging)"
      mask help: Speedgoat Driver Block<br>IO336-325k - IO336 Analog setup<br><br>&copy; 2007 - 2026, Speedgoat GmbH, <a href="matlab: web('www.speedgoat.com','-browser');">www.speedgoat.com</a>
      mask init:
      | p = sg_fpga_io336_analog_setup_m.runMaskInit(); %#ok<NASGU>
      settings: OpenFcn=sg_fpga_io336_analog_setup_m.runOpenMaskCb();
      mask Help: eval('sg.utils.help.show(''io_main/refentry_io336_analog_setup_v1'');')
      mask TypeOptions id: 1 | 2 | 3 | 4 | 5 | 6 | 7 | 8 | 9 | 10
      mask Callback id: sg_fpga_io336_analog_setup_m.runModuleIdCb();
      mask Callback parEnableCodeModule1: sg_fpga_io336_analog_setup_m.runEnableCmCb(1);
      mask Callback parEnableCodeModule2: sg_fpga_io336_analog_setup_m.runEnableCmCb(2);
      mask Callback parEnableCodeModule3: sg_fpga_io336_analog_setup_m.runEnableCmCb(3);
      mask Callback parEnableCodeModule4: sg_fpga_io336_analog_setup_m.runEnableCmCb(4);
      mask Callback parEnableCodeModule5: sg_fpga_io336_analog_setup_m.runEnableCmCb(5);
      mask Callback parEnableCodeModule6: sg_fpga_io336_analog_setup_m.runEnableCmCb(6);
      mask Callback parEnableCodeModule7: sg_fpga_io336_analog_setup_m.runEnableCmCb(7);
      mask Callback parEnableCodeModule8: sg_fpga_io336_analog_setup_m.runEnableCmCb(8);
      mask Callback parAdcEnableIndividualTrigger: sg_fpga_io336_analog_setup_m.runAnalogInputCb();
      mask TypeOptions parAdcTriggerMode1: Model Step | I/O Module Clock | I/O Module Internal Signal | I/O Module Digital I/O
      mask Callback parAdcTriggerMode1: sg_fpga_io336_analog_setup_m.runAdcTriggerCb('suffix', '1')
      mask TypeOptions parAdcInternalTrigger1: <empty>
      mask TypeOptions parAdcOversampling1: None | 2 | 4 | 8 | 16 | 32 | 64
      mask TypeOptions parAdcTriggerMode2: Model Step | I/O Module Clock | I/O Module Internal Signal | I/O Module Digital I/O
      mask Callback parAdcTriggerMode2: sg_fpga_io336_analog_setup_m.runAdcTriggerCb('suffix', '2')
      mask TypeOptions parAdcInternalTrigger2: <empty>
      mask TypeOptions parAdcOversampling2: None | 2 | 4 | 8 | 16 | 32 | 64
      mask Callback parAdcEnableFrame: sg_fpga_io336_analog_setup_m.runEnableFrameCb();
      mask TypeOptions parAdcTriggerMode: Model Step | I/O Module Clock | I/O Module Internal Signal | I/O Module Digital I/O
      mask Callback parAdcTriggerMode: sg_fpga_io336_analog_setup_m.runAdcTriggerCb();
      mask TypeOptions parAdcInternalTrigger: <empty>
      mask TypeOptions parAdcOversampling: None | 2 | 4 | 8 | 16 | 32 | 64
      mask TypeOptions parDacTriggerMode: Model Step | I/O Module Clock | I/O Module Internal Signal | I/O Module Digital I/O
      mask Callback parDacTriggerMode: sg_fpga_io336_analog_setup_m.runDacTriggerCb();
      mask TypeOptions parDacInternalTrigger: <empty>
      mask Callback parDacEnableFrame: sg_fpga_io336_analog_setup_m.runDacTriggerCb();
      mask Callback dacUsesTimer: sg_fpga_io336_analog_setup_m.runDacTriggerCb();
      mask Callback parAdcChannel1: sg_fpga_io336_analog_setup_m.runAnalogInputCb();
      mask Callback parAdcChannel2: sg_fpga_io336_analog_setup_m.runAnalogInputCb();
      mask Callback parAdcChannel3: sg_fpga_io336_analog_setup_m.runAnalogInputCb();
      mask Callback parAdcChannel4: sg_fpga_io336_analog_setup_m.runAnalogInputCb();
      mask Callback parAdcChannel5: sg_fpga_io336_analog_setup_m.runAnalogInputCb();
      mask Callback parAdcChannel6: sg_fpga_io336_analog_setup_m.runAnalogInputCb();
      mask Callback parAdcChannel7: sg_fpga_io336_analog_setup_m.runAnalogInputCb();
      mask Callback parAdcChannel8: sg_fpga_io336_analog_setup_m.runAnalogInputCb();
      mask Callback parVoltageRangePerChannelEn1: sg_fpga_io336_analog_setup_m.runAnalogInputCb();
      mask TypeOptions parAdcRangeAll1: +/- 20V | +/- 10V | +/- 5V
      mask TypeOptions parAdcRange1: +/- 20V | +/- 10V | +/- 5V
      mask TypeOptions parAdcRange3: +/- 20V | +/- 10V | +/- 5V
      mask TypeOptions parAdcRange2: +/- 20V | +/- 10V | +/- 5V
      mask TypeOptions parAdcRange4: +/- 20V | +/- 10V | +/- 5V
      mask Callback parAdcChannel9: sg_fpga_io336_analog_setup_m.runAnalogInputCb();
      mask Callback parAdcChannel10: sg_fpga_io336_analog_setup_m.runAnalogInputCb();
      mask Callback parAdcChannel11: sg_fpga_io336_analog_setup_m.runAnalogInputCb();
      mask Callback parAdcChannel12: sg_fpga_io336_analog_setup_m.runAnalogInputCb();
      mask Callback parAdcChannel13: sg_fpga_io336_analog_setup_m.runAnalogInputCb();
      mask Callback parAdcChannel14: sg_fpga_io336_analog_setup_m.runAnalogInputCb();
      mask Callback parAdcChannel15: sg_fpga_io336_analog_setup_m.runAnalogInputCb();
      mask Callback parAdcChannel16: sg_fpga_io336_analog_setup_m.runAnalogInputCb();
      mask Callback parVoltageRangePerChannelEn2: sg_fpga_io336_analog_setup_m.runAnalogInputCb();
      mask TypeOptions parAdcRangeAll2: +/- 20V | +/- 10V | +/- 5V
      mask TypeOptions parAdcRange5: +/- 20V | +/- 10V | +/- 5V
      mask TypeOptions parAdcRange7: +/- 20V | +/- 10V | +/- 5V
      mask TypeOptions parAdcRange6: +/- 20V | +/- 10V | +/- 5V
      mask TypeOptions parAdcRange8: +/- 20V | +/- 10V | +/- 5V
      mask Callback parDacChannel1: sg_fpga_io336_analog_setup_m.runAnalogOutputCb();
      mask Callback parDacChannel2: sg_fpga_io336_analog_setup_m.runAnalogOutputCb();
      mask Callback parDacChannel3: sg_fpga_io336_analog_setup_m.runAnalogOutputCb();
      mask Callback parDacChannel4: sg_fpga_io336_analog_setup_m.runAnalogOutputCb();
      mask Callback parDacChannel5: sg_fpga_io336_analog_setup_m.runAnalogOutputCb();
      mask Callback parDacChannel6: sg_fpga_io336_analog_setup_m.runAnalogOutputCb();
      mask Callback parDacChannel7: sg_fpga_io336_analog_setup_m.runAnalogOutputCb();
      mask Callback parDacChannel8: sg_fpga_io336_analog_setup_m.runAnalogOutputCb();
      mask TypeOptions parDacRange1: +-2.5 V | +-5 V | +-10 V
      mask TypeOptions parDacRange2: +-2.5 V | +-5 V | +-10 V
      mask TypeOptions parDacRange3: +-2.5 V | +-5 V | +-10 V
      mask TypeOptions parDacRange4: +-2.5 V | +-5 V | +-10 V
      mask TypeOptions parDacRange5: +-2.5 V | +-5 V | +-10 V
      mask TypeOptions parDacRange6: +-2.5 V | +-5 V | +-10 V
      mask TypeOptions parDacRange7: +-2.5 V | +-5 V | +-10 V
      mask TypeOptions parDacRange8: +-2.5 V | +-5 V | +-10 V
      mask DialogControl tabMain Prompt: Main
      mask DialogControl boxModuleSettings Prompt: Module Settings
      mask DialogControl boxCodeModules Prompt: Code Module Functionality
      mask DialogControl boxAdcTrigger Prompt: Analog Input Trigger
      mask DialogControl boxAdcIndividualTrigger Prompt: Individual Trigger Settings (Sample Based)
      mask DialogControl boxAdcTrigger1 Prompt: Channel 01-08
      mask DialogControl boxAdcTrigger2 Prompt: Channel 09-16
      mask DialogControl boxAdcCommonTrigger Prompt: Common Trigger Settings
      mask DialogControl boxAdcFrameSettings Prompt: Frame-Based Settings
      mask DialogControl parAdcTriggerResolutionInfo Prompt: placeholder
      mask DialogControl parAdcSampleRateFrameInfo Prompt:
      | => 100 kHz
      | (10 us/sample)
      mask DialogControl parAdcFrameSizeInfo Prompt: => 100
      mask DialogControl parAdcSampleTimeInfo Prompt: => 1 ms
      mask DialogControl boxDacTrigger Prompt: Analog Output Trigger
      mask DialogControl boxDacFrameSettings Prompt: Frame-Based Settings
      mask DialogControl parDacFifoThresholdInfo Prompt: placeholder
      mask DialogControl parDacTriggerResolutionInfo Prompt: placeholder
      mask DialogControl parDacSampleRateInfo Prompt:
      | => 1 MHz
      | (1 us/sample)
      mask DialogControl parDacFrameSizeInfo Prompt: => 1000
      mask DialogControl parDacSampleTimeInfo Prompt: => 1 ms
      mask DialogControl tabAdc Prompt: Analog Inputs
      mask DialogControl boxAdc1 Prompt: Channel 01-08
      mask DialogControl parAdcAvailableChannels1 Prompt: Available Channels
      mask DialogControl VoltageRangeBox1 Prompt: Individual voltage range
      mask DialogControl boxAdc2 Prompt: Channel 09-16
      mask DialogControl parAdcAvailableChannels2 Prompt: Available Channels
      mask DialogControl VoltageRangeBox2 Prompt: Individual voltage range
      mask DialogControl tabDac Prompt: Analog Outputs
      mask DialogControl boxDacSetting Prompt: Channel Settings
      mask DialogControl boxDacChannels Prompt: Available Channels
      mask DialogControl boxDacChannel1 Prompt: Channel 1
      mask DialogControl boxDacChannel2 Prompt: Channel 2
      mask DialogControl boxDacChannel3 Prompt: Channel 3
      mask DialogControl boxDacChannel4 Prompt: Channel 4
      mask DialogControl boxDacChannel5 Prompt: Channel 5
      mask DialogControl boxDacChannel6 Prompt: Channel 6
      mask DialogControl boxDacChannel7 Prompt: Channel 7
      mask DialogControl boxDacChannel8 Prompt: Channel 8
      mask Display: disp('Speedgoat\nIO336-325k\nAnalog setup v1\nModule ID: 1');
